simulink library "yoshi"  (R2013b)
settings: Solver=ode45  StartTime=0.0  StopTime=10.0  RelTol=1e-3
undefined symbols (not defined in the file): DiscIntNeverNeededParam, K, R
libraries: legonxtlib x3
settings Model: Creator=grouleau  LastModifiedBy=abhayg

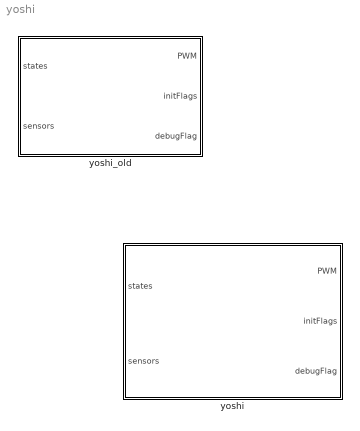
== system yoshi ==
  yoshi : Stateflow chart  TreatAsAtomicUnit=on
      settings: CopyFcn=set_param(gcbh, 'DSMNames', '', 'DSMValues', '', 'CopyFcn', '')
  yoshi_old : Stateflow chart  TreatAsAtomicUnit=on

== system yoshi/yoshi/Yoshi.Speak ==
  f : TriggerPort  TriggerType=function-call
      settings: CopyFcn=Stateflow.SLINSF.SimulinkMan.removeBlockPreDeleteFcn  PreDeleteFcn=Stateflow.SLINSF.SimulinkMan.unsafePredeleteFcn
  Constant : Constant  Value=50
  Speaker : legonxtlib/Speaker  sinputMode=Volume only  sspeakerFreq=800  sspeakerVolume=50  sspeakerDuration=100
  wires:
  Constant/1 -> Speaker/1

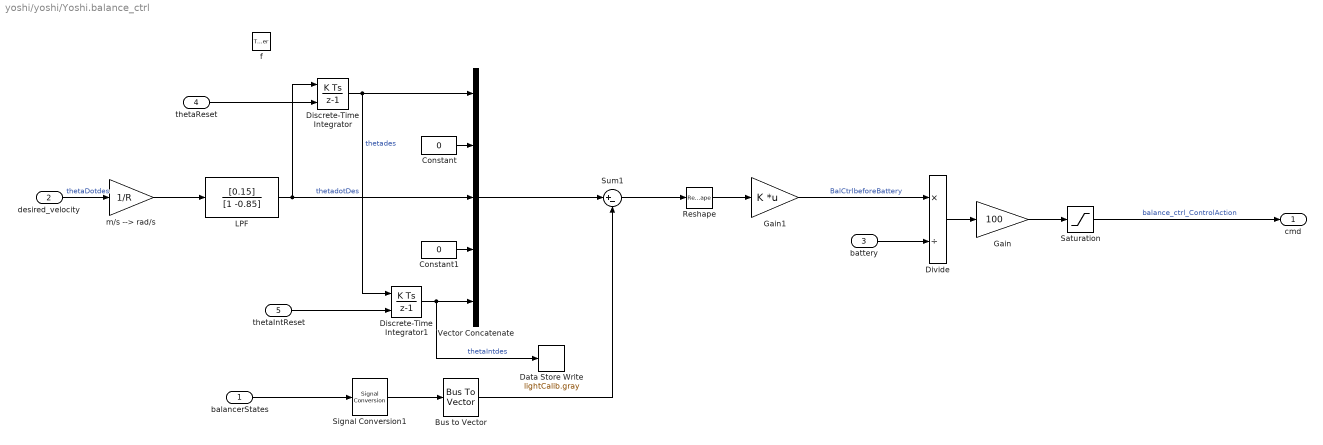
== system yoshi/yoshi/Yoshi.balance_ctrl ==
  balancerStates : Inport  OutDataTypeStr=Bus: Balancer_States_Bus  PortDimensions=1
  desired_velocity : Inport  Port=2  OutDataTypeStr=single  PortDimensions=1  BusOutputAsStruct=on
  battery : Inport  Port=3  OutDataTypeStr=double  PortDimensions=1
  thetaReset : Inport  Port=4  OutDataTypeStr=single  PortDimensions=1  BusOutputAsStruct=on
  thetaIntReset : Inport  Port=5  OutDataTypeStr=single  PortDimensions=1  BusOutputAsStruct=on
  f : TriggerPort  TriggerType=function-call
      settings: CopyFcn=Stateflow.SLINSF.SimulinkMan.removeBlockPreDeleteFcn  PreDeleteFcn=Stateflow.SLINSF.SimulinkMan.unsafePredeleteFcn
  Bus to Vector : BusToVector
  Constant : Constant  Value=0  OutDataTypeStr=single
  Constant1 : Constant  Value=0  OutDataTypeStr=single
  Data Store Write : DataStoreWrite  DataStoreName=lightCalib  DataStoreElements=lightCalib.gray
  Discrete-Time Integrator : DiscreteIntegrator  ExternalReset=rising  SampleTime=-1  ICPrevOutput=DiscIntNeverNeededParam  ICPrevScaledInput=DiscIntNeverNeededParam
  Discrete-Time Integrator1 : DiscreteIntegrator  ExternalReset=rising  SampleTime=-1  ICPrevOutput=DiscIntNeverNeededParam  ICPrevScaledInput=DiscIntNeverNeededParam
  Divide : Product  Inputs=*/
  Gain : Gain  Gain=100
  Gain1 : Gain  Gain=K  Multiplication=Matrix(K*u)
  LPF : DiscreteFilter  Numerator=[0.15]  Denominator=[1 -0.85]
  Reshape : Reshape  OutputDimensionality=Column vector (2-D)
  Saturation : Saturate  UpperLimit=100  LowerLimit=-100  OutDataTypeStr=single
  Signal Conversion1 : SignalConversion  ConversionOutput=Virtual bus
  Sum1 : Sum  Inputs=|+-
  Vector Concatenate : Concatenate  NumInputs=5
  m/s --> rad/s : Gain  Gain=1/R
  cmd : Outport  OutDataTypeStr=single  PortDimensions=1  InitialOutput=0
  wires:
  Discrete-Time Integrator1/1 -> Data Store Write/1, Vector Concatenate/5  "thetaIntdes"
  Discrete-Time Integrator/1 -> Vector Concatenate/1, Discrete-Time Integrator1/1  "thetades"
  Constant1/1 -> Vector Concatenate/4
  LPF/1 -> Vector Concatenate/3, Discrete-Time Integrator/1  "thetadotDes"
  Constant/1 -> Vector Concatenate/2
  m/s --> rad/s/1 -> LPF/1
  Signal Conversion1/1 -> Bus to Vector/1
  Divide/1 -> Gain/1
  Gain/1 -> Saturation/1
  Gain1/1 -> Divide/1  "BalCtrlbeforeBattery"
  Saturation/1 -> cmd/1  "balance_ctrl_ControlAction"
  battery/1 -> Divide/2
  Vector Concatenate/1 -> Sum1/1
  balancerStates/1 -> Signal Conversion1/1
  Bus to Vector/1 -> Sum1/2
  desired_velocity/1 -> m/s --> rad/s/1  "thetaDotdes"
  Sum1/1 -> Reshape/1
  Reshape/1 -> Gain1/1
  thetaReset/1 -> Discrete-Time Integrator/2
  thetaIntReset/1 -> Discrete-Time Integrator1/2

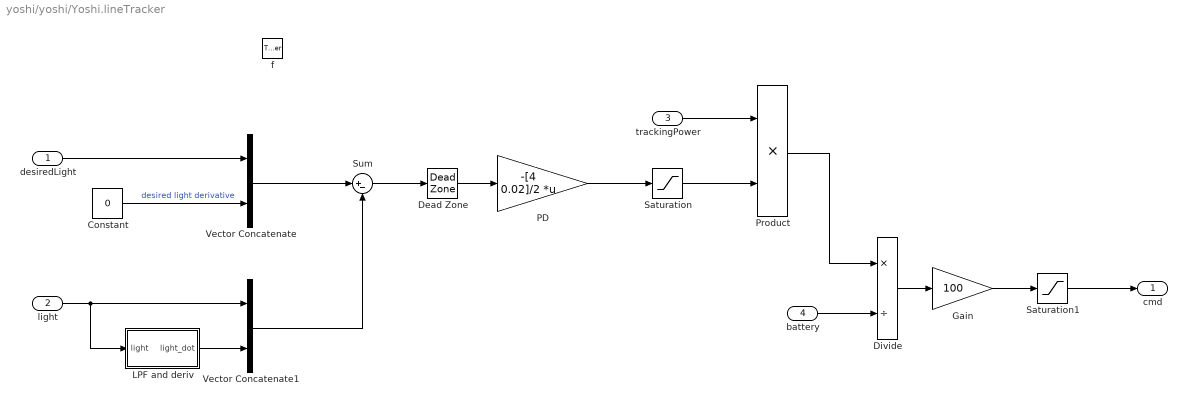
== system yoshi/yoshi/Yoshi.lineTracker ==
  desiredLight : Inport  OutDataTypeStr=single  PortDimensions=1
  light : Inport  Port=2  OutDataTypeStr=single  PortDimensions=1
  trackingPower : Inport  Port=3  OutDataTypeStr=single  PortDimensions=1
  battery : Inport  Port=4  OutDataTypeStr=double  PortDimensions=1
  f : TriggerPort  TriggerType=function-call
      settings: CopyFcn=Stateflow.SLINSF.SimulinkMan.removeBlockPreDeleteFcn  PreDeleteFcn=Stateflow.SLINSF.SimulinkMan.unsafePredeleteFcn
  Constant : Constant  Value=0  OutDataTypeStr=single
  Dead Zone : DeadZone  LowerValue=-0.02  UpperValue=0.02  SaturateOnIntegerOverflow=on
  Divide : Product  Inputs=*/
  Gain : Gain  Gain=100
  LPF and deriv : Subsystem
  PD : Gain  Gain="-[4  0.02]/2"  Multiplication=Matrix(K*u)
  Product : Product
  Saturation : Saturate  UpperLimit=6  LowerLimit=-6
  Saturation1 : Saturate  UpperLimit=100  LowerLimit=-100  OutDataTypeStr=single
  Sum : Sum  Inputs=|+-
  Vector Concatenate : Concatenate
  Vector Concatenate1 : Concatenate
  cmd : Outport  OutDataTypeStr=single  PortDimensions=1
  wires:
  Divide/1 -> Gain/1
  Gain/1 -> Saturation1/1
  battery/1 -> Divide/2
  Saturation1/1 -> cmd/1
  Product/1 -> Divide/1
  trackingPower/1 -> Product/1
  Saturation/1 -> Product/2
  PD/1 -> Saturation/1
  Dead Zone/1 -> PD/1
  Sum/1 -> Dead Zone/1
  Vector Concatenate1/1 -> Sum/2
  Vector Concatenate/1 -> Sum/1
  light/1 -> Vector Concatenate1/1, LPF and deriv/1(light)
  LPF and deriv/1(light_dot) -> Vector Concatenate1/2
  Constant/1 -> Vector Concatenate/2  "desired light derivative"
  desiredLight/1 -> Vector Concatenate/1

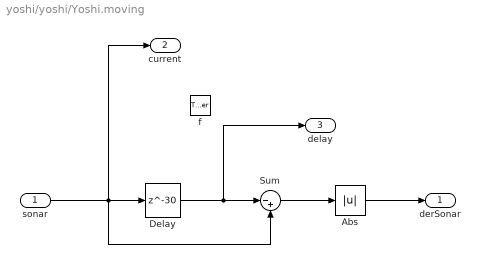
== system yoshi/yoshi/Yoshi.moving ==
  sonar : Inport  OutDataTypeStr=single  PortDimensions=1
  f : TriggerPort  TriggerType=function-call
      settings: CopyFcn=Stateflow.SLINSF.SimulinkMan.removeBlockPreDeleteFcn  PreDeleteFcn=Stateflow.SLINSF.SimulinkMan.unsafePredeleteFcn
  Abs : Abs
  Delay : Delay  DelayLength=30  InitialCondition=0
  Sum : Sum  Inputs=|-+
  derSonar : Outport  OutDataTypeStr=single
  current : Outport  Port=2  OutDataTypeStr=single
  delay : Outport  Port=3  OutDataTypeStr=single
  wires:
  Delay/1 -> delay/1, Sum/1
  sonar/1 -> current/1, Sum/2, Delay/1
  Sum/1 -> Abs/1
  Abs/1 -> derSonar/1

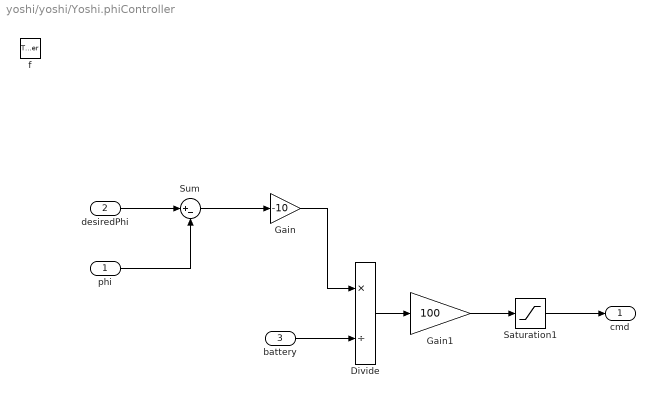
== system yoshi/yoshi/Yoshi.phiController ==
  phi : Inport  OutDataTypeStr=single  PortDimensions=1
  desiredPhi : Inport  Port=2  OutDataTypeStr=single  PortDimensions=1
  battery : Inport  Port=3  OutDataTypeStr=double  PortDimensions=1
  f : TriggerPort  TriggerType=function-call
      settings: CopyFcn=Stateflow.SLINSF.SimulinkMan.removeBlockPreDeleteFcn  PreDeleteFcn=Stateflow.SLINSF.SimulinkMan.unsafePredeleteFcn
  Divide : Product  Inputs=*/
  Gain : Gain  Gain=-10
  Gain1 : Gain  Gain=100
  Saturation1 : Saturate  UpperLimit=100  LowerLimit=-100  OutDataTypeStr=single
  Sum : Sum  Inputs=|+-
  cmd : Outport
  wires:
  Saturation1/1 -> cmd/1
  Gain/1 -> Divide/1
  Divide/1 -> Gain1/1
  Gain1/1 -> Saturation1/1
  battery/1 -> Divide/2
  Sum/1 -> Gain/1
  phi/1 -> Sum/2
  desiredPhi/1 -> Sum/1

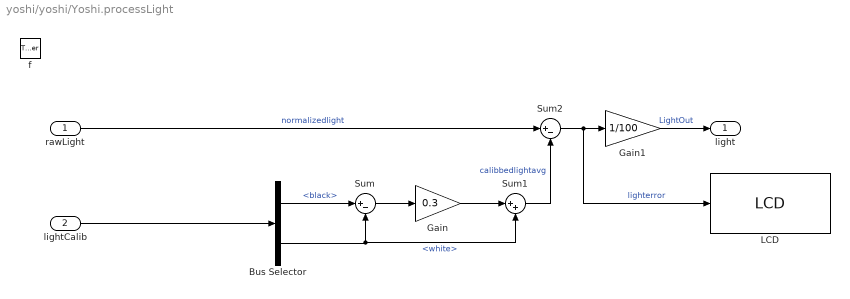
== system yoshi/yoshi/Yoshi.processLight ==
  rawLight : Inport  OutDataTypeStr=single  PortDimensions=1
  lightCalib : Inport  Port=2  OutDataTypeStr=Bus: Light_Bus  PortDimensions=1
  f : TriggerPort  TriggerType=function-call
      settings: CopyFcn=Stateflow.SLINSF.SimulinkMan.removeBlockPreDeleteFcn  PreDeleteFcn=Stateflow.SLINSF.SimulinkMan.unsafePredeleteFcn
  Bus Selector : BusSelector  OutputSignals=black,white
  Gain : Gain  Gain=0.3
  Gain1 : Gain  Gain=1/100
  LCD : legonxtlib/LCD  slcdStr=Light  slcdLine=2  slcdFormat=Decimal
  Sum : Sum  Inputs=|+-
  Sum1 : Sum  Inputs=|++
  Sum2 : Sum  Inputs=|+-
  light : Outport
  wires:
  Gain1/1 -> light/1  "LightOut"
  Sum2/1 -> LCD/1, Gain1/1  "lighterror"
  Sum1/1 -> Sum2/2  "calibbedlightavg"
  rawLight/1 -> Sum2/1  "normalizedlight"
  Gain/1 -> Sum1/1
  Sum/1 -> Gain/1
  Bus Selector/2 -> Sum/2, Sum1/2  "<white>"
  Bus Selector/1 -> Sum/1  "<black>"
  lightCalib/1 -> Bus Selector/1

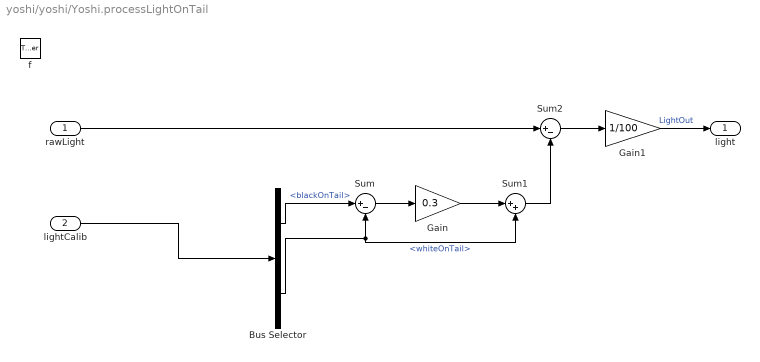
== system yoshi/yoshi/Yoshi.processLightOnTail ==
  rawLight : Inport  OutDataTypeStr=single  PortDimensions=1
  lightCalib : Inport  Port=2  OutDataTypeStr=Bus: Light_Bus  PortDimensions=1
  f : TriggerPort  TriggerType=function-call
      settings: CopyFcn=Stateflow.SLINSF.SimulinkMan.removeBlockPreDeleteFcn  PreDeleteFcn=Stateflow.SLINSF.SimulinkMan.unsafePredeleteFcn
  Bus Selector : BusSelector  OutputSignals=blackOnTail,whiteOnTail
  Gain : Gain  Gain=0.3
  Gain1 : Gain  Gain=1/100
  Sum : Sum  Inputs=|+-
  Sum1 : Sum  Inputs=|++
  Sum2 : Sum  Inputs=|+-
  light : Outport
  wires:
  Gain1/1 -> light/1  "LightOut"
  Sum2/1 -> Gain1/1
  Sum1/1 -> Sum2/2
  rawLight/1 -> Sum2/1
  Gain/1 -> Sum1/1
  Sum/1 -> Gain/1
  Bus Selector/2 -> Sum/2, Sum1/2  "<whiteOnTail>"
  Bus Selector/1 -> Sum/1  "<blackOnTail>"
  lightCalib/1 -> Bus Selector/1

== system yoshi/yoshi/Yoshi.tail_controller ==
  note: Could be improved, PI for example
  current : Inport  OutDataTypeStr=single  PortDimensions=1
  desired : Inport  Port=2  OutDataTypeStr=single  PortDimensions=1
  f : TriggerPort  TriggerType=function-call
      settings: CopyFcn=Stateflow.SLINSF.SimulinkMan.removeBlockPreDeleteFcn  PreDeleteFcn=Stateflow.SLINSF.SimulinkMan.unsafePredeleteFcn
  Gain : Gain  Gain=250
  Saturation : Saturate  UpperLimit=100  LowerLimit=-100  OutDataTypeStr=single
  Sum : Sum  Inputs=|+-
  cmd : Outport  OutDataTypeStr=single  PortDimensions=1  InitialOutput=0
  wires:
  Saturation/1 -> cmd/1
  Gain/1 -> Saturation/1
  desired/1 -> Sum/1
  current/1 -> Sum/2
  Sum/1 -> Gain/1

== system yoshi/yoshi_old/see_saw_mode.Speak ==
  f : TriggerPort  TriggerType=function-call
      settings: CopyFcn=Stateflow.SLINSF.SimulinkMan.removeBlockPreDeleteFcn  PreDeleteFcn=Stateflow.SLINSF.SimulinkMan.unsafePredeleteFcn
  Constant : Constant  Value=50
  Speaker : legonxtlib/Speaker  sinputMode=Volume only  sspeakerFreq=800  sspeakerVolume=50  sspeakerDuration=100
  wires:
  Constant/1 -> Speaker/1

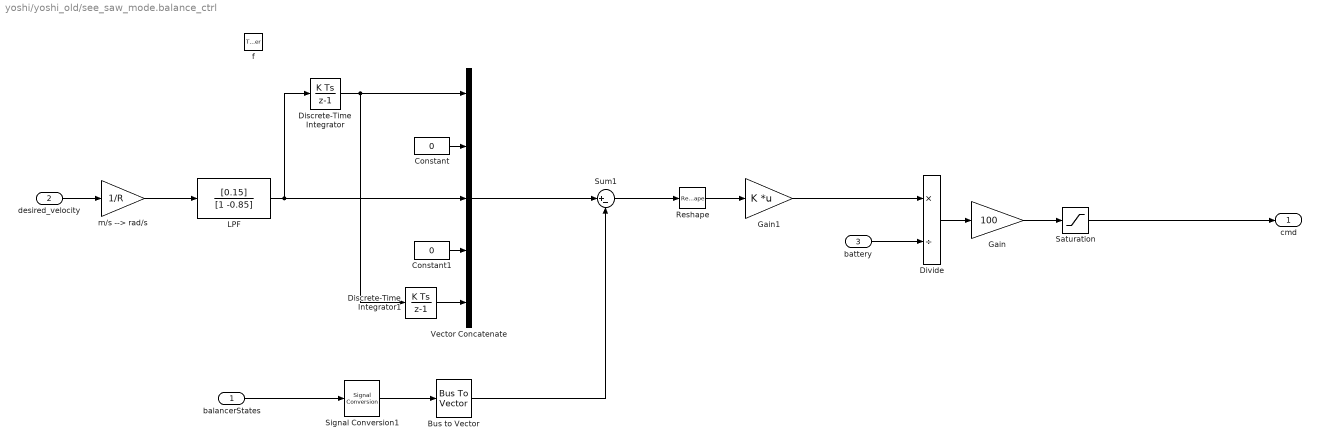
== system yoshi/yoshi_old/see_saw_mode.balance_ctrl ==
  balancerStates : Inport  OutDataTypeStr=Bus: Balancer_States_Bus  PortDimensions=1
  desired_velocity : Inport  Port=2  OutDataTypeStr=single  PortDimensions=1  BusOutputAsStruct=on
  battery : Inport  Port=3  OutDataTypeStr=double  PortDimensions=1
  f : TriggerPort  TriggerType=function-call
      settings: CopyFcn=Stateflow.SLINSF.SimulinkMan.removeBlockPreDeleteFcn  PreDeleteFcn=Stateflow.SLINSF.SimulinkMan.unsafePredeleteFcn
  Bus to Vector : BusToVector
  Constant : Constant  Value=0  OutDataTypeStr=single
  Constant1 : Constant  Value=0  OutDataTypeStr=single
  Discrete-Time Integrator : DiscreteIntegrator  SampleTime=-1  ICPrevOutput=DiscIntNeverNeededParam  ICPrevScaledInput=DiscIntNeverNeededParam
  Discrete-Time Integrator1 : DiscreteIntegrator  SampleTime=-1  ICPrevOutput=DiscIntNeverNeededParam  ICPrevScaledInput=DiscIntNeverNeededParam
  Divide : Product  Inputs=*/
  Gain : Gain  Gain=100
  Gain1 : Gain  Gain=K  Multiplication=Matrix(K*u)
  LPF : DiscreteFilter  Numerator=[0.15]  Denominator=[1 -0.85]
  Reshape : Reshape  OutputDimensionality=Column vector (2-D)
  Saturation : Saturate  UpperLimit=100  LowerLimit=-100  OutDataTypeStr=single
  Signal Conversion1 : SignalConversion  ConversionOutput=Virtual bus
  Sum1 : Sum  Inputs=|+-
  Vector Concatenate : Concatenate  NumInputs=5
  m/s --> rad/s : Gain  Gain=1/R
  cmd : Outport  OutDataTypeStr=single  PortDimensions=1  InitialOutput=0
  wires:
  Discrete-Time Integrator1/1 -> Vector Concatenate/5
  Discrete-Time Integrator/1 -> Vector Concatenate/1, Discrete-Time Integrator1/1
  Constant1/1 -> Vector Concatenate/4
  LPF/1 -> Vector Concatenate/3, Discrete-Time Integrator/1
  Constant/1 -> Vector Concatenate/2
  m/s --> rad/s/1 -> LPF/1
  Signal Conversion1/1 -> Bus to Vector/1
  Divide/1 -> Gain/1
  Gain/1 -> Saturation/1
  Gain1/1 -> Divide/1
  Saturation/1 -> cmd/1
  battery/1 -> Divide/2
  Vector Concatenate/1 -> Sum1/1
  balancerStates/1 -> Signal Conversion1/1
  Bus to Vector/1 -> Sum1/2
  desired_velocity/1 -> m/s --> rad/s/1
  Sum1/1 -> Reshape/1
  Reshape/1 -> Gain1/1

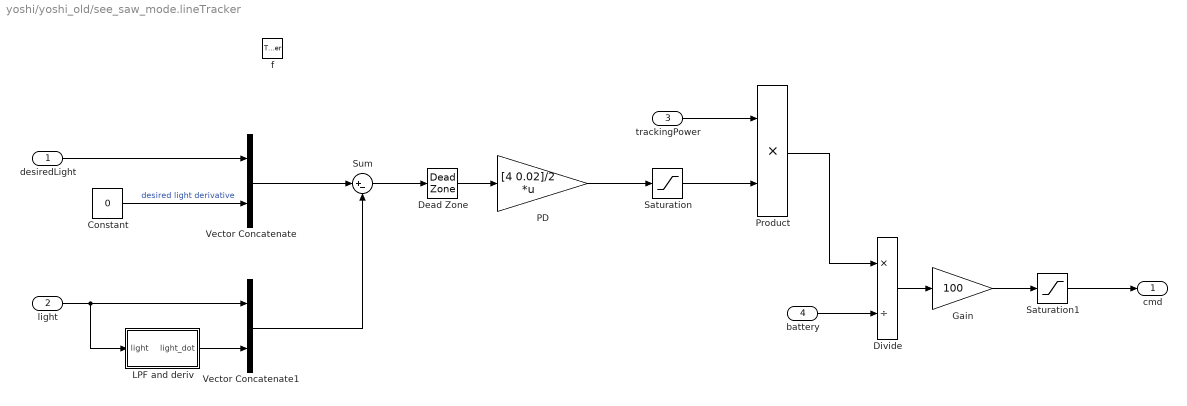
== system yoshi/yoshi_old/see_saw_mode.lineTracker ==
  desiredLight : Inport  OutDataTypeStr=single  PortDimensions=1
  light : Inport  Port=2  OutDataTypeStr=single  PortDimensions=1
  trackingPower : Inport  Port=3  OutDataTypeStr=single  PortDimensions=1
  battery : Inport  Port=4  OutDataTypeStr=double  PortDimensions=1
  f : TriggerPort  TriggerType=function-call
      settings: CopyFcn=Stateflow.SLINSF.SimulinkMan.removeBlockPreDeleteFcn  PreDeleteFcn=Stateflow.SLINSF.SimulinkMan.unsafePredeleteFcn
  Constant : Constant  Value=0  OutDataTypeStr=single
  Dead Zone : DeadZone  LowerValue=-0.02  UpperValue=0.02  SaturateOnIntegerOverflow=on
  Divide : Product  Inputs=*/
  Gain : Gain  Gain=100
  LPF and deriv : Subsystem
  PD : Gain  Gain="[4  0.02]/2"  Multiplication=Matrix(K*u)
  Product : Product
  Saturation : Saturate  UpperLimit=6  LowerLimit=-6
  Saturation1 : Saturate  UpperLimit=100  LowerLimit=-100  OutDataTypeStr=single
  Sum : Sum  Inputs=|+-
  Vector Concatenate : Concatenate
  Vector Concatenate1 : Concatenate
  cmd : Outport  OutDataTypeStr=single  PortDimensions=1
  wires:
  Divide/1 -> Gain/1
  Gain/1 -> Saturation1/1
  battery/1 -> Divide/2
  Saturation1/1 -> cmd/1
  Product/1 -> Divide/1
  trackingPower/1 -> Product/1
  Saturation/1 -> Product/2
  PD/1 -> Saturation/1
  Dead Zone/1 -> PD/1
  Sum/1 -> Dead Zone/1
  Vector Concatenate1/1 -> Sum/2
  Vector Concatenate/1 -> Sum/1
  light/1 -> Vector Concatenate1/1, LPF and deriv/1(light)
  LPF and deriv/1(light_dot) -> Vector Concatenate1/2
  Constant/1 -> Vector Concatenate/2  "desired light derivative"
  desiredLight/1 -> Vector Concatenate/1

== system yoshi/yoshi_old/see_saw_mode.moving ==
  sonar : Inport  OutDataTypeStr=single  PortDimensions=1
  f : TriggerPort  TriggerType=function-call
      settings: CopyFcn=Stateflow.SLINSF.SimulinkMan.removeBlockPreDeleteFcn  PreDeleteFcn=Stateflow.SLINSF.SimulinkMan.unsafePredeleteFcn
  Abs : Abs
  Delay : Delay  DelayLength=30  InitialCondition=0
  Sum : Sum  Inputs=|-+
  derSonar : Outport  OutDataTypeStr=single
  current : Outport  Port=2  OutDataTypeStr=single
  delay : Outport  Port=3  OutDataTypeStr=single
  wires:
  Delay/1 -> delay/1, Sum/1
  sonar/1 -> current/1, Sum/2, Delay/1
  Sum/1 -> Abs/1
  Abs/1 -> derSonar/1

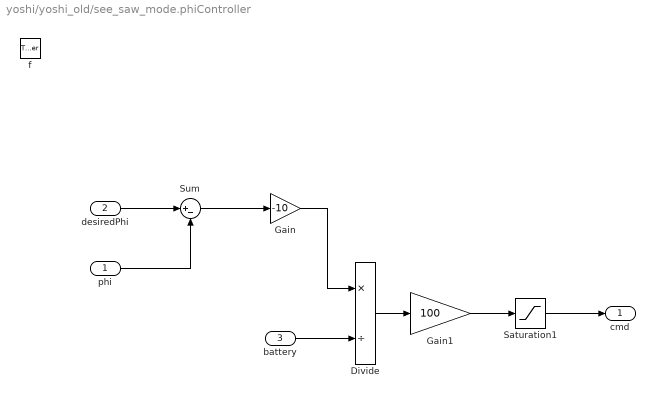
== system yoshi/yoshi_old/see_saw_mode.phiController ==
  phi : Inport  OutDataTypeStr=single  PortDimensions=1
  desiredPhi : Inport  Port=2  OutDataTypeStr=single  PortDimensions=1
  battery : Inport  Port=3  OutDataTypeStr=double  PortDimensions=1
  f : TriggerPort  TriggerType=function-call
      settings: CopyFcn=Stateflow.SLINSF.SimulinkMan.removeBlockPreDeleteFcn  PreDeleteFcn=Stateflow.SLINSF.SimulinkMan.unsafePredeleteFcn
  Divide : Product  Inputs=*/
  Gain : Gain  Gain=-10
  Gain1 : Gain  Gain=100
  Saturation1 : Saturate  UpperLimit=100  LowerLimit=-100  OutDataTypeStr=single
  Sum : Sum  Inputs=|+-
  cmd : Outport
  wires:
  Saturation1/1 -> cmd/1
  Gain/1 -> Divide/1
  Divide/1 -> Gain1/1
  Gain1/1 -> Saturation1/1
  battery/1 -> Divide/2
  Sum/1 -> Gain/1
  phi/1 -> Sum/2
  desiredPhi/1 -> Sum/1

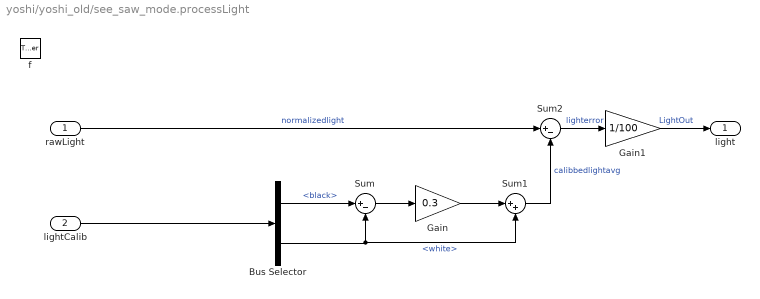
== system yoshi/yoshi_old/see_saw_mode.processLight ==
  rawLight : Inport  OutDataTypeStr=single  PortDimensions=1
  lightCalib : Inport  Port=2  OutDataTypeStr=Bus: Light_Bus  PortDimensions=1
  f : TriggerPort  TriggerType=function-call
      settings: CopyFcn=Stateflow.SLINSF.SimulinkMan.removeBlockPreDeleteFcn  PreDeleteFcn=Stateflow.SLINSF.SimulinkMan.unsafePredeleteFcn
  Bus Selector : BusSelector  OutputSignals=black,white
  Gain : Gain  Gain=0.3
  Gain1 : Gain  Gain=1/100
  Sum : Sum  Inputs=|+-
  Sum1 : Sum  Inputs=|++
  Sum2 : Sum  Inputs=|+-
  light : Outport
  wires:
  Gain1/1 -> light/1  "LightOut"
  Sum2/1 -> Gain1/1  "lighterror"
  Sum1/1 -> Sum2/2  "calibbedlightavg"
  rawLight/1 -> Sum2/1  "normalizedlight"
  Gain/1 -> Sum1/1
  Sum/1 -> Gain/1
  Bus Selector/2 -> Sum/2, Sum1/2  "<white>"
  Bus Selector/1 -> Sum/1  "<black>"
  lightCalib/1 -> Bus Selector/1

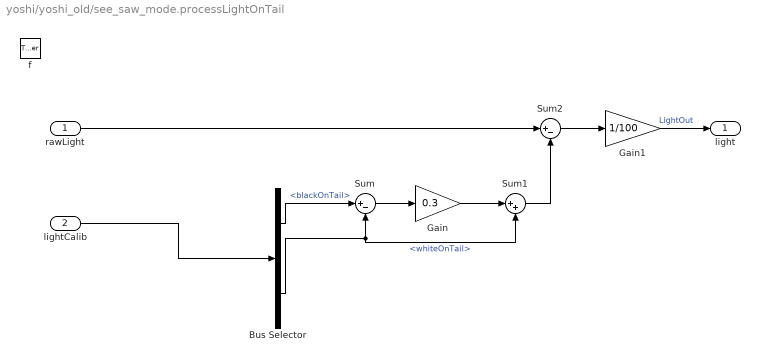
== system yoshi/yoshi_old/see_saw_mode.processLightOnTail ==
  rawLight : Inport  OutDataTypeStr=single  PortDimensions=1
  lightCalib : Inport  Port=2  OutDataTypeStr=Bus: Light_Bus  PortDimensions=1
  f : TriggerPort  TriggerType=function-call
      settings: CopyFcn=Stateflow.SLINSF.SimulinkMan.removeBlockPreDeleteFcn  PreDeleteFcn=Stateflow.SLINSF.SimulinkMan.unsafePredeleteFcn
  Bus Selector : BusSelector  OutputSignals=blackOnTail,whiteOnTail
  Gain : Gain  Gain=0.3
  Gain1 : Gain  Gain=1/100
  Sum : Sum  Inputs=|+-
  Sum1 : Sum  Inputs=|++
  Sum2 : Sum  Inputs=|+-
  light : Outport
  wires:
  Gain1/1 -> light/1  "LightOut"
  Sum2/1 -> Gain1/1
  Sum1/1 -> Sum2/2
  rawLight/1 -> Sum2/1
  Gain/1 -> Sum1/1
  Sum/1 -> Gain/1
  Bus Selector/2 -> Sum/2, Sum1/2  "<whiteOnTail>"
  Bus Selector/1 -> Sum/1  "<blackOnTail>"
  lightCalib/1 -> Bus Selector/1

== system yoshi/yoshi_old/see_saw_mode.tail_controller ==
  note: Could be improved, PI for example
  current : Inport  OutDataTypeStr=single  PortDimensions=1
  desired : Inport  Port=2  OutDataTypeStr=single  PortDimensions=1
  f : TriggerPort  TriggerType=function-call
      settings: CopyFcn=Stateflow.SLINSF.SimulinkMan.removeBlockPreDeleteFcn  PreDeleteFcn=Stateflow.SLINSF.SimulinkMan.unsafePredeleteFcn
  Gain : Gain  Gain=250
  Saturation : Saturate  UpperLimit=100  LowerLimit=-100  OutDataTypeStr=single
  Sum : Sum  Inputs=|+-
  cmd : Outport  OutDataTypeStr=single  PortDimensions=1  InitialOutput=0
  wires:
  Saturation/1 -> cmd/1
  Gain/1 -> Saturation/1
  desired/1 -> Sum/1
  current/1 -> Sum/2
  Sum/1 -> Gain/1

== system yoshi/yoshi/Yoshi.lineTracker/LPF and deriv ==
  light : Inport
  Discrete Filter : DiscreteFilter  Numerator=[0.05]  Denominator=[1 -0.95]
  Gain : Gain  Gain=1/0.004
  Sum3 : Sum  Inputs=+-
  Unit Delay : UnitDelay  SampleTime=-1
  light_dot : Outport
  wires:
  Unit Delay/1 -> Sum3/2
  Gain/1 -> Unit Delay/1, Sum3/1
  Sum3/1 -> light_dot/1  "theta_dot_dot"
  Discrete Filter/1 -> Gain/1
  light/1 -> Discrete Filter/1

== system yoshi/yoshi_old/see_saw_mode.lineTracker/LPF and deriv ==
  light : Inport
  Discrete Filter : DiscreteFilter  Numerator=[0.05]  Denominator=[1 -0.95]
  Gain : Gain  Gain=1/0.004
  Sum3 : Sum  Inputs=+-
  Unit Delay : UnitDelay  SampleTime=-1
  light_dot : Outport
  wires:
  Unit Delay/1 -> Sum3/2
  Gain/1 -> Unit Delay/1, Sum3/1
  Sum3/1 -> light_dot/1  "theta_dot_dot"
  Discrete Filter/1 -> Gain/1
  light/1 -> Discrete Filter/1

== stateflow chart yoshi/yoshi ==
  state Yoshi
    entry:
    desired_tail = single(1.6);
    des_light_ramp_up = single(0.3);
    des_light_ramp_down = single(0.7);
    during:
    normalizedLight = processLight(sensors.light,lightCalib);
    normalizedLightOnRamp = processLightOnTail(sensors.light,lightCalib)
    PWM.tail = tail_controller(sensors.theta_T, desired_tail);
    state Pause
      entry:
      debugFlag = uint16(601);
    state light = processLight(rawLight,lightCalib) [function]
    state StandUp
      entry: debugFlag = uint16(602);
      initFlags.theta = single(1);
      initFlags.gyroReset = single(1);
      during:
      desired_tail = desired_tail + single(0.0008);
    state light = processLightOnTail(rawLight,lightCalib) [function]
    state Balancing
      state SeesawLogic [parallel]
        settings: executionOrder=1
        state StationnaryBalance
          entry: debugFlag = uint16(6031);
          desired_tail = single(0);
          initFlags.theta = single(0);
          initFlags.gyroReset = single(0);
          desired_states = balancerStates_Bus0;
        state ApproachRamp
          entry: debugFlag = uint16(604);
          during:
          state CheckIfRampHasBeenHit
            entry:
            counter=single(0);
            turningPWM = lineTracker(single(0), normalizedLight, single(1), sensors.battery);
            during:
            if(states.balancerStates.theta_dot<=0)
            counter = counter + single(1);
            else
            counter = single(0);
            end
            turningPWM = lineTracker(single(0), normalizedLight, single(1), sensors.battery);
            exit:
            Speak;
            phi_desired=states.phi;
            theta_temp=states.balancerStates.theta;
          state StartWalking
            entry:
            debugFlag = uint16(605);
            turningPWM = lineTracker(single(0), normalizedLight, single(1), sensors.battery);
            %des_vel = single(0.04);
            during:
            des_vel = des_vel+single(0.00024);
            turningPWM = lineTracker(single(0), normalizedLight, single(1), sensors.battery);
          state PushOverTheRRamp
            entry:
            debugFlag=uint16(712)
            des_vel=single(0.15);
            during:
            turningPWM=phiController(states.phi,phi_desired, sensors.battery);
            des_vel=single(0.15);
          (default) -> StartWalking
          StartWalking -> CheckIfRampHasBeenHit : [des_vel >= single(0.1)]
          CheckIfRampHasBeenHit -> PushOverTheRRamp : [counter>=single(10)]
        state Slowdown2
          entry:
          theta_temp=states.balancerStates.theta;
          en,du:
          des_vel=des_vel-single(0.00012);
          turningPWM = single(2)*lineTracker(des_light_ramp_up, normalizedLight, single(1), sensors.battery) + phiController(states.phi,phi_desired, sensors.battery);
        state WalkUpRamp %Putting both phiControl & lineTrack+phiControl states in one. Simple if-else statement
          entry:
          debugFlag=uint16(1011)
          en,du,ex:
          des_vel=single(0.08);
          turningPWM = single(2)*lineTracker(des_light_ramp_up, normalizedLight, single(1), sensors.battery) + phiController(states.phi,phi_desired, sensors.battery);
        state Slowdown
          entry:
          Speak;
          theta_temp=states.balancerStates.theta;
          en,du,ex:
          des_vel=des_vel-single(0.00012);
          turningPWM = single(2)*lineTracker(des_light_ramp_up, normalizedLight, single(1), sensors.battery) + phiController(states.phi,phi_desired, sensors.battery);
        state StopAndBalanceOverYoshi
          state FallDetectionCheck
            entry:
            Speak;
            during:
            turningPWM =single(2)*lineTracker(single(0.4), normalizedLight, single(1), sensors.battery) + phiController(states.phi,phi_desired, sensors.battery);
            des_vel=single(0.04);
            exit:
            des_vel=single(0.0);
          state ResetThetaAndControlAction
            entry:
            Speak
            debugFlag=uint16(45);
            during:
            turningPWM = phiController(states.phi,phi_desired, sensors.battery);
            des_vel = single(0);
          (default) -> FallDetectionCheck
          FallDetectionCheck -> ResetThetaAndControlAction : [states.balancerStates.theta-theta_temp>3.25*3.14] %1.5 rotations after we get on the ramp
        state Sonar2
          entry:
          debugFlag = uint16(604);
          note: 
          state YoshiIsMoving
            entry:
            des_vel=single(0);
            during:
            turningPWM = phiController(states.phi,phi_desired, sensors.battery);
            des_vel = single(0);
            turningPWM = phiController(states.phi,phi_desired, sensors.battery);
          state AreWeMoving
            entry:
            des_vel=single(0);
            turningPWM = phiController(states.phi,phi_desired, sensors.battery);
            debugFlag=uint16(111)
            [derSonar,Curr,Delay2]=moving(sensors.sonar)
          state keepchcking
            entry:
            des_vel=single(0);
            numTimes = numTimes+1;
            turningPWM = phiController(states.phi,phi_desired, sensors.battery);
            exit:
            theta_temp=states.balancerStates.theta;
          state WalkOffRover
            entry:
            theta_temp=states.balancerStates.theta;
            debugFlag = uint16(6011);
            des_vel = single(0.01);
            turningPWM = single(2)*lineTracker(des_light_ramp_down, normalizedLight, single(1), sensors.battery)+single(0.5)*phiController(states.phi,phi_desired, sensors.battery); ;
            during:
            turningPWM = single(2)*lineTracker(des_light_ramp_down, normalizedLight, single(1), sensors.battery)+single(0.5)*phiController(states.phi,phi_desired, sensors.battery); ;
            if (des_vel<single(0.1))
            des_vel = des_vel+single(0.00024);
            else des_vel=single(0.1);
            end
          state SlowDownOffRamp
            entry:
            Speak
            debugFlag = uint16(6012);
            des_vel = des_vel-single(0.00024);
            turningPWM = lineTracker(single(0), normalizedLight, single(1), sensors.battery) ;
            during:
            turningPWM = lineTracker(single(0), normalizedLight, single(1), sensors.battery);
            des_vel = des_vel-single(0.00024);
            exit:
            phi_desired=states.phi;
          state StopAndPassControl
            entry: debugFlag = uint16(6013);
            des_vel=single(0.04);
            turningPWM = lineTracker(single(0), normalizedLight, single(1), sensors.battery);
          YoshiIsMoving -> AreWeMoving : [sensors.sonar<40]
          AreWeMoving -> YoshiIsMoving [order 1] : [sensors.sonar>100]
          (junction 351) -> AreWeMoving [order 1] : [derSonar>single(10)]{numTimes=0;}
          AreWeMoving -> (junction 351) [order 2] : %default
          (junction 351) -> keepchcking [order 2]
          keepchcking -> AreWeMoving [order 1]
          (default) -> WalkOffRover
          keepchcking -> ? [order 1] : [numTimes>(20*10)]
          WalkOffRover -> SlowDownOffRamp : [states.balancerStates.theta-theta_temp>single(6*3.14)] % 3.5 rotations
          SlowDownOffRamp -> StopAndPassControl : [des_vel<=single(0.04)]
        state RaceDone
          en,du: debugFlag = uint16(599);
          des_vel=single(0.06);
          forwardPWM = balance_ctrl(states.balancerStates, des_vel ,sensors.battery,single(0),single(0))
          turningPWM = lineTracker(single(0), normalizedLight, single(1), sensors.battery);
          current_mode_status = OperationModeStatusEnum.SUCCESSFULLY_COMPLETED;
        (default) -> StationnaryBalance
        StationnaryBalance -> ApproachRamp : after(2,sec)
        PushOverTheRRamp -> Slowdown2 : [states.balancerStates.theta-theta_temp>single(1.57/2)]{counter=single(0);}
        Slowdown2 -> WalkUpRamp %Putting both phiControl & lineTrack+phiControl states in one. Simple if-else statement : [des_vel<=single(0.08)]
        WalkUpRamp %Putting both phiControl & lineTrack+phiControl states in one. Simple if-else statement -> Slowdown : [states.balancerStates.theta-theta_temp>3.5*3.14] %1.5 rotations after we get on the ramp
        Slowdown -> StopAndBalanceOverYoshi : [des_vel <= single(0.04)]
        StopAndPassControl -> RaceDone : after(1,tick)
        ResetThetaAndControlAction -> Sonar2 : [sensors.BT_status_in==single(StatusID.NXT1_GO_DOWN_RAMP) || after(6,sec)]
      state After [parallel]
        during:
        forwardPWM = balance_ctrl(states.balancerStates, des_vel ,sensors.battery,single(0),single(0))
        PWM.left = forwardPWM + turningPWM;
        PWM.right = forwardPWM -turningPWM;
        settings: executionOrder=2
    state [derSonar,current,delay] = moving(sonar) [function]
    state cmd = phiController(phi,desiredPhi,battery) [function]
    state cmd = lineTracker(desiredLight,light,trackingPower,battery) [function]
    state Speak [function]
    state cmd = tail_controller(current,desired) [function]
    state cmd = balance_ctrl(balancerStates,desired_velocity,battery,thetaReset,thetaIntReset) [function]
    (default) -> Pause
    Pause -> StandUp
    StandUp -> Balancing : [desired_tail >=single(2.0) && sensors.theta_T >= single(2.0)]
  note: ?
  data: rawLight function_input single size=1; lightCalib function_input Bus: Light_Bus size=1; light function_output; rawLight function_input single size=1; lightCalib function_input Bus: Light_Bus size=1; light function_output; sonar function_input single size=1; derSonar function_output single; current function_output single; delay function_output single; cmd function_output; phi function_input single size=1; desiredPhi function_input single size=1; battery function_input double size=1; cmd function_output single size=1; desiredLight function_input single size=1; light function_input single size=1; trackingPower function_input single size=1; battery function_input double size=1; current function_input single size=1; desired function_input single size=1; cmd function_output single size=1; balancerStates function_input Bus: Balancer_States_Bus size=1; desired_velocity function_input single size=1; battery function_input double size=1; cmd function_output single size=1; thetaReset function_input single size=1; thetaIntReset function_input single size=1; states input Bus: States_Bus size=1; sensors input Bus: Sensors_Bus size=1; PWM output Bus: PWM_bus size=1; initFlags output Bus: Init_Bus size=1; debugFlag output uint16 size=1; desired_states local Bus: Balancer_States_Bus size=1; desired_tail local single size=1; current_mode_status data_store_memory; balancerStates_Bus0 parameter Bus: Balancer_States_Bus size=1; lightCalib data_store_memory; normalizedLight local single size=1; des_vel local single size=1; theta_ref local single size=1; forwardPWM local single size=1; turningPWM local single size=1; BT_status_out local single size=1; desired_phi local single size=1; phi0 local single size=1; Curr local; Delay2 local; derSonar local; numTimes local; normalizedLightOnRamp local; phi_desired local; counter local; chart2 local; counter2 local; theta_temp local single; des_light_ramp_down local; des_light_ramp_up local

== stateflow chart yoshi/yoshi_old ==
  state see_saw_mode
    entry:
    desired_tail = single(1.6);
    during:
    normalizedLight = processLight(sensors.light,lightCalib);
    normalizedLightOnRamp = processLightOnTail(sensors.light,lightCalib)
    PWM.tail = tail_controller(sensors.theta_T, desired_tail);
    state Pause
      entry:
      debugFlag = uint16(601);
    state light = processLight(rawLight,lightCalib) [function]
    state StandUp
      entry: debugFlag = uint16(602);
      initFlags.theta = single(1);
      initFlags.gyroReset = single(1);
      during:
      desired_tail = desired_tail + single(0.0008);
    state light = processLightOnTail(rawLight,lightCalib) [function]
    state Balancing
      state SeesawLogic [parallel]
        settings: executionOrder=1
        state StationnaryBalance
          entry: debugFlag = uint16(603);
          desired_tail = single(0.5);
          initFlags.theta = single(0);
          initFlags.gyroReset = single(0);
          desired_states = balancerStates_Bus0;
        state ApproachRamp
          entry: debugFlag = uint16(604);
          during:
          turningPWM = lineTracker(single(0), normalizedLight, single(1), sensors.battery);
          state StartWalking
            entry:
            entry: debugFlag = uint16(605);
            des_vel = single(0.04);
            during:
            des_vel = des_vel+single(0.00024);
            Speak;
          state CheckIfRampHasBeenHit
            entry:
            counter=single(0);
            during:
            if(states.balancerStates.theta_dot<=0)
            counter = counter + single(1);
            else
            counter = single(0);
            end
          state HitTheRamp
            entry:
            counter2=single(0);
            Speak
            exit:
            phi_desired=states.phi;
          (default) -> StartWalking
          StartWalking -> CheckIfRampHasBeenHit : [des_vel >= single(0.1)]
          CheckIfRampHasBeenHit -> HitTheRamp : [counter>=single(10)]
        state WalkUpRamp %Putting both phiControl & lineTrack+phiControl states in one. Simple if-else statement
          entry:
          des_vel=single(0.05);
          turningPWM = lineTracker(single(0), normalizedLight, single(1), sensors.battery) + phiController(states.phi,phi_desired, sensors.battery);
          debugFlag = uint16(1);
          during:
          des_vel=single(0.05);
          turningPWM = lineTracker(single(0), normalizedLight, single(1), sensors.battery) + phiController(states.phi,phi_desired, sensors.battery);
          debugFlag = uint16(2);
          exit:
          des_vel=single(0.05);
          turningPWM = lineTracker(single(0), normalizedLight, single(1), sensors.battery) + phiController(states.phi,phi_desired, sensors.battery);
        state FallDetectionCheck %Need to update criteria
          during:
          turningPWM = lineTracker(single(0), normalizedLight, single(1), sensors.battery) + phiController(states.phi,phi_desired, sensors.battery);
          des_vel=single(0.05);
          if(states.balancerStates.theta_dot>single(5))
          counter=counter+single(1);
          debugFlag=uint16(2);
          elseif(states.balancerStates.theta_dot<single(2))
          counter=single(0);
          debugFlag=uint16(3);
          end
          exit:
          turningPWM = lineTracker(single(0), normalizedLight, single(1), sensors.battery) + phiController(states.phi,phi_desired, sensors.battery);
          des_vel=single(0.05);
        state GetReadytoStop
          entry:
          debugFlag=uint16(4);
          Speak
          during:
          turningPWM = lineTracker(single(0), normalizedLight, single(1), sensors.battery) + phiController(states.phi,phi_desired, sensors.battery);
          des_vel = des_vel-single(0.00012);
        state StopOverYoshi
          entry:
          debugFlag = uint16(5);
          des_vel = des_vel-single(0.00012);
          phi_desired=states.phi;
          Speak
          during: %do I need to copy this to 'entry'?
          des_vel = des_vel-single(0.00012);
          turningPWM = phiController(states.phi,phi_desired, sensors.battery);
        state Stop
          entry:
          des_vel=single(0);
          turningPWM = phiController(states.phi,phi_desired, sensors.battery);
          during:
          des_vel=single(0);
          turningPWM = phiController(states.phi,phi_desired, sensors.battery);
        state Sonar2
          entry: debugFlag = uint16(604);
          during:
          turningPWM = lineTracker(single(0), normalizedLight, single(1), sensors.battery);
          exit:
          turningPWM = single(0);
          note: 
          state YoshiIsMoving
            during: des_vel = single(0.0005);
          state AreWeMoving
            entry:
            debugFlag=uint16(111)
            [derSonar,Curr,Delay2]=moving(sensors.sonar)
          state keepchcking
            entry:
            numTimes = numTimes+1;
          state WalkOffRover
            entry:
            entry: debugFlag = uint16(6011);
            des_vel = single(0.01);
            during:
            des_vel = des_vel+single(0.00024);
          (default) -> YoshiIsMoving
          AreWeMoving -> YoshiIsMoving [order 1] : [sensors.sonar>100]
          YoshiIsMoving -> AreWeMoving : [sensors.sonar<40]
          (junction 397) -> AreWeMoving [order 1] : [derSonar>4]{numTimes=0;}
          AreWeMoving -> (junction 397) [order 2] : %default
          (junction 397) -> keepchcking [order 2]
          keepchcking -> AreWeMoving [order 2]
          keepchcking -> WalkOffRover [order 1] : [numTimes>(20*25)]
        state RaceDone
          entry: debugFlag = uint16(599);
          current_mode_status = OperationModeStatusEnum.SUCCESSFULLY_COMPLETED;
        (default) -> StationnaryBalance
        StationnaryBalance -> ApproachRamp : after(5,sec)
        HitTheRamp -> WalkUpRamp %Putting both phiControl & lineTrack+phiControl states in one. Simple if-else statement : [after(0.5,sec)]{counter=single(0);}
        WalkUpRamp %Putting both phiControl & lineTrack+phiControl states in one. Simple if-else statement -> FallDetectionCheck %Need to update criteria : after(5,sec)
        FallDetectionCheck %Need to update criteria -> GetReadytoStop : [counter>=single(20)]
        GetReadytoStop -> StopOverYoshi : after(1,sec)
        StopOverYoshi -> Stop : [des_vel<=single(0)]
        Stop -> Sonar2 : after(5,sec)
      state After [parallel]
        during:
        forwardPWM = balance_ctrl(states.balancerStates, des_vel ,sensors.battery)
        PWM.left = forwardPWM + turningPWM;
        PWM.right = forwardPWM - turningPWM;
        settings: executionOrder=2
    state [derSonar,current,delay] = moving(sonar) [function]
    state cmd = phiController(phi,desiredPhi,battery) [function]
    state cmd = lineTracker(desiredLight,light,trackingPower,battery) [function]
    state Speak [function]
    state cmd = tail_controller(current,desired) [function]
    state cmd = balance_ctrl(balancerStates,desired_velocity,battery) [function]
    (default) -> Pause
    Pause -> StandUp : after(3,sec)
    StandUp -> Balancing : [desired_tail >=single(2.0) && sensors.theta_T >= single(2.0)]
  data: rawLight function_input single size=1; lightCalib function_input Bus: Light_Bus size=1; light function_output; rawLight function_input single size=1; lightCalib function_input Bus: Light_Bus size=1; light function_output; sonar function_input single size=1; derSonar function_output single; current function_output single; delay function_output single; cmd function_output; phi function_input single size=1; desiredPhi function_input single size=1; battery function_input double size=1; cmd function_output single size=1; desiredLight function_input single size=1; light function_input single size=1; trackingPower function_input single size=1; battery function_input double size=1; current function_input single size=1; desired function_input single size=1; cmd function_output single size=1; balancerStates function_input Bus: Balancer_States_Bus size=1; desired_velocity function_input single size=1; battery function_input double size=1; cmd function_output single size=1; states input Bus: States_Bus size=1; sensors input Bus: Sensors_Bus size=1; PWM output Bus: PWM_bus size=1; initFlags output Bus: Init_Bus size=1; debugFlag output uint16 size=1; desired_states local Bus: Balancer_States_Bus size=1; desired_tail local single size=1; current_mode_status data_store_memory; balancerStates_Bus0 parameter Bus: Balancer_States_Bus size=1; lightCalib data_store_memory; normalizedLight local single size=1; des_vel local single size=1; forwardPWM local single size=1; turningPWM local single size=1; Curr local; Delay2 local; derSonar local; numTimes local; normalizedLightOnRamp local; phi_desired local; counter local; counter2 local
